simulink subsystem "EMS_sim"  (R2023b)
settings: Solver=VariableStepAuto  StartTime=0.0  StopTime=10.0  RelTol=1e-3
undefined symbols (not defined in the file or in its folder): CH, EMS, Ts
settings Model: Creator=ortolud16324  LastModifiedBy=ortolud16324

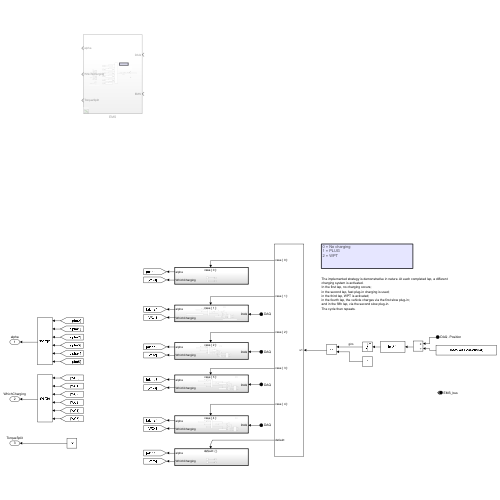
[thumbnail: Simulink's stored preview of the top-level diagram]
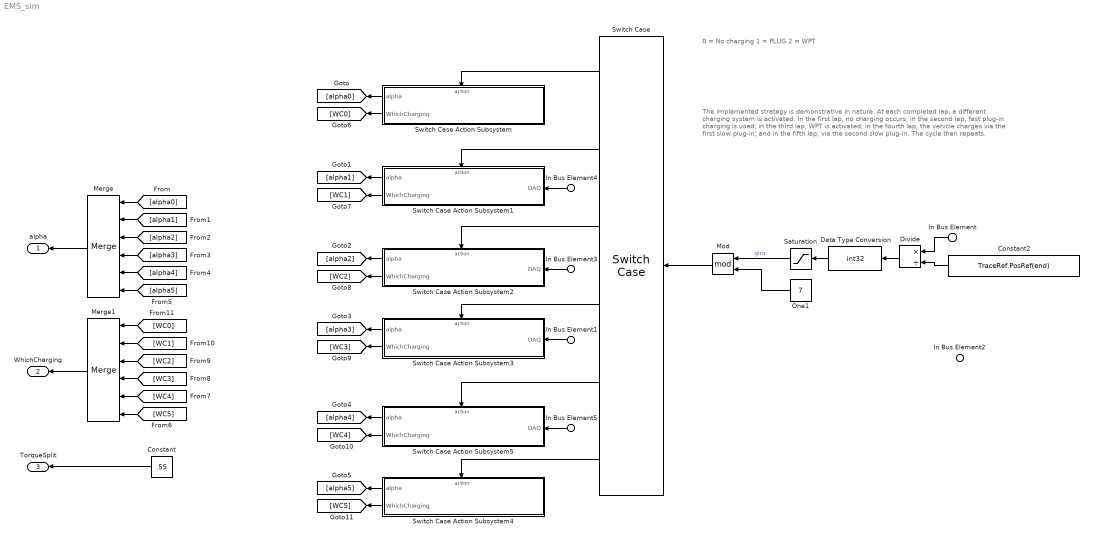
== system EMS_sim ==
  note: 0 = No charging
      | 1 = PLUG
      | 2 = WPT
  note: The implemented strategy is demonstrative in nature. At each completed lap, a different charging system is activated.
      | In the first lap, no charging occurs;
      | in the second lap, fast plug-in charging is used;
      | in the third lap, WPT is activated;
      | in the fourth lap, the vehicle charges via the first slow plug-in;
      | and in the fifth lap, via the second slow plug-in.
      | The cycle then repeats.
  In Bus Element{1,3..5} (4 alike) : Inport  PortName=DAQ
  In Bus Element : Inport  PortName=DAQ  Element=Position
  In Bus Element2 : Inport  Port=2  PortName=EMS_bus
  Constant : Constant  Value=.55  SampleTime=Ts
  Constant2 : Constant  Value=TraceRef.PosRef(end)
  Data Type Conversion : DataTypeConversion  OutDataTypeStr=int32  SaturateOnIntegerOverflow=off  RndMeth=Floor
  Divide : Product  Inputs=*/
  Merge : Merge  Inputs=6
  Merge1 : Merge  Inputs=6
  Mod : Math  Operator=mod
  One1 : Constant  Value=7  OutDataTypeStr=Inherit: Inherit via back propagation
  Saturation : Saturate  UpperLimit=100000  LowerLimit=0
  Switch Case : SwitchCase  CaseConditions={0,1,2,3,4}
  Switch Case Action Subsystem : Subsystem  TreatAsAtomicUnit=on
  Switch Case Action Subsystem1 : Subsystem  TreatAsAtomicUnit=on
  Switch Case Action Subsystem2 : Subsystem  TreatAsAtomicUnit=on
  Switch Case Action Subsystem3 : Subsystem  TreatAsAtomicUnit=on
  Switch Case Action Subsystem4 : Subsystem  TreatAsAtomicUnit=on
  Switch Case Action Subsystem5 : Subsystem  TreatAsAtomicUnit=on
  alpha : Outport
  WhichCharging : Outport  Port=2
  TorqueSplit : Outport  Port=3
  wires:
  Merge1/1 -> WhichCharging/1
  Constant/1 -> TorqueSplit/1
  Merge/1 -> alpha/1
  [alpha2] -> Merge/3
  Switch Case Action Subsystem2/2(WhichCharging) -> [WC2]
  [alpha3] -> Merge/4
  [WC3] -> Merge1/4
  [WC5] -> Merge1/6
  [WC4] -> Merge1/5
  [WC1] -> Merge1/2
  [WC2] -> Merge1/3
  One1/1 -> Mod/2
  In Bus Element5/1 -> Switch Case Action Subsystem5/1(DAQ)
  Switch Case Action Subsystem5/2(WhichCharging) -> [WC4]
  Switch Case/5 -> Switch Case Action Subsystem5/Action
  Switch Case/6 -> Switch Case Action Subsystem4/Action
  [alpha4] -> Merge/5
  Switch Case Action Subsystem2/1(alpha) -> [alpha2]
  Switch Case Action Subsystem3/2(WhichCharging) -> [WC3]
  [alpha0] -> Merge/1
  Switch Case Action Subsystem1/2(WhichCharging) -> [WC1]
  In Bus Element1/1 -> Switch Case Action Subsystem3/1(DAQ)
  Switch Case Action Subsystem5/1(alpha) -> [alpha4]
  Switch Case Action Subsystem3/1(alpha) -> [alpha3]
  Switch Case Action Subsystem/2(WhichCharging) -> [WC0]
  [alpha1] -> Merge/2
  In Bus Element4/1 -> Switch Case Action Subsystem1/1(DAQ)
  Switch Case Action Subsystem/1(alpha) -> [alpha0]
  Switch Case Action Subsystem1/1(alpha) -> [alpha1]
  Switch Case Action Subsystem4/1(alpha) -> [alpha5]
  Data Type Conversion/1 -> Saturation/1
  Mod/1 -> Switch Case/1
  In Bus Element3/1 -> Switch Case Action Subsystem2/1(DAQ)
  Switch Case/4 -> Switch Case Action Subsystem3/Action
  Switch Case/2 -> Switch Case Action Subsystem1/Action
  Switch Case/1 -> Switch Case Action Subsystem/Action
  Divide/1 -> Data Type Conversion/1
  [WC0] -> Merge1/1
  Constant2/1 -> Divide/2
  In Bus Element/1 -> Divide/1
  Saturation/1 -> Mod/1  "giro"
  Switch Case Action Subsystem4/2(WhichCharging) -> [WC5]
  Switch Case/3 -> Switch Case Action Subsystem2/Action
  [alpha5] -> Merge/6

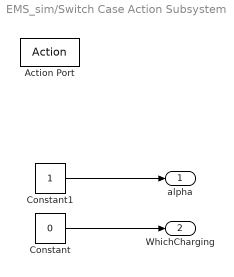
== system EMS_sim/Switch Case Action Subsystem ==
  Action Port : ActionPort
  Constant : Constant  Value=0
  Constant1 : Constant
  alpha : Outport
  WhichCharging : Outport  Port=2
  wires:
  Constant/1 -> WhichCharging/1
  Constant1/1 -> alpha/1

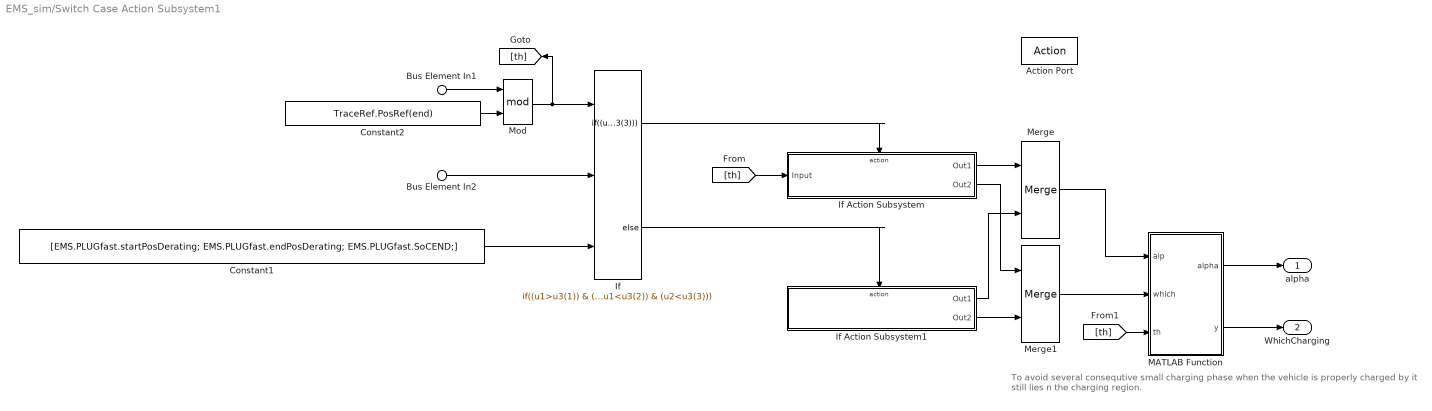
== system EMS_sim/Switch Case Action Subsystem1 ==
  note: To avoid several consequtive small charging phase when the vehicle is properly charged by it still lies n the charging region.
  Bus Element In1 : Inport  PortName=DAQ  Element=Position
  Bus Element In2 : Inport  PortName=DAQ  Element=SoC_BP
  Action Port : ActionPort
  Constant1 : Constant  Value=[EMS.PLUGfast.startPosDerating; EMS.PLUGfast.endPosDerating; EMS.PLUGfast.SoCEND;]
  Constant2 : Constant  Value=TraceRef.PosRef(end)
  If : If  NumInputs=3  IfExpression=(u1>u3(1)) & (u1<u3(2)) & (u2<u3(3))
  If Action Subsystem : Subsystem  TreatAsAtomicUnit=on
  If Action Subsystem1 : Subsystem  TreatAsAtomicUnit=on
  MATLAB Function : MATLAB Function  TreatAsAtomicUnit=on
  Merge : Merge
  Merge1 : Merge
  Mod : Math  Operator=mod
  alpha : Outport
  WhichCharging : Outport  Port=2
  wires:
  Merge/1 -> MATLAB Function/1(alp)
  Merge1/1 -> MATLAB Function/2(which)
  If/1 -> If Action Subsystem/Action
  If/2 -> If Action Subsystem1/Action
  Constant2/1 -> Mod/2
  If Action Subsystem/1(Out1) -> Merge/1
  If Action Subsystem1/1(Out1) -> Merge/2
  Mod/1 -> [th], If/1
  Bus Element In1/1 -> Mod/1
  Bus Element In2/1 -> If/2
  Constant1/1 -> If/3
  If Action Subsystem/2(Out2) -> Merge1/1
  If Action Subsystem1/2(Out2) -> Merge1/2
  [th] -> If Action Subsystem/1(Input)
  MATLAB Function/2(y) -> WhichCharging/1
  [th] -> MATLAB Function/3(th)
  MATLAB Function/1(alpha) -> alpha/1

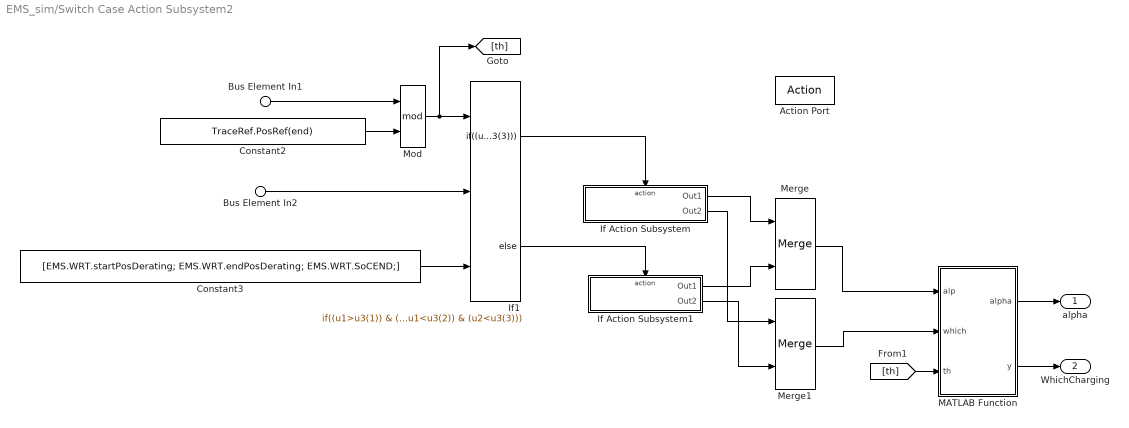
== system EMS_sim/Switch Case Action Subsystem2 ==
  Bus Element In1 : Inport  PortName=DAQ  Element=Position
  Bus Element In2 : Inport  PortName=DAQ  Element=SoC_BP
  Action Port : ActionPort
  Constant2 : Constant  Value=TraceRef.PosRef(end)
  Constant3 : Constant  Value=[EMS.WRT.startPosDerating; EMS.WRT.endPosDerating; EMS.WRT.SoCEND;]
  If Action Subsystem : Subsystem  TreatAsAtomicUnit=on
  If Action Subsystem1 : Subsystem  TreatAsAtomicUnit=on
  If1 : If  NumInputs=3  IfExpression=(u1>u3(1)) & (u1<u3(2)) & (u2<u3(3))
  MATLAB Function : MATLAB Function  TreatAsAtomicUnit=on
  Merge : Merge
  Merge1 : Merge
  Mod : Math  Operator=mod
  alpha : Outport
  WhichCharging : Outport  Port=2
  wires:
  Constant2/1 -> Mod/2
  Mod/1 -> [th], If1/1
  Bus Element In1/1 -> Mod/1
  If1/1 -> If Action Subsystem/Action
  If1/2 -> If Action Subsystem1/Action
  If Action Subsystem/1(Out1) -> Merge/1
  If Action Subsystem1/1(Out1) -> Merge/2
  If Action Subsystem/2(Out2) -> Merge1/1
  If Action Subsystem1/2(Out2) -> Merge1/2
  Bus Element In2/1 -> If1/2
  Constant3/1 -> If1/3
  Merge/1 -> MATLAB Function/1(alp)
  Merge1/1 -> MATLAB Function/2(which)
  [th] -> MATLAB Function/3(th)
  MATLAB Function/1(alpha) -> alpha/1
  MATLAB Function/2(y) -> WhichCharging/1

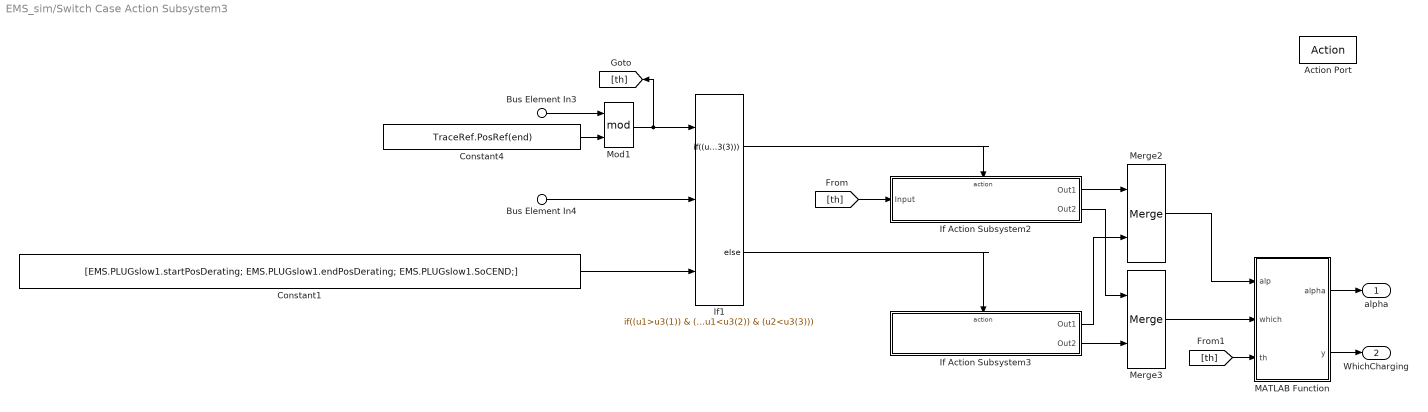
== system EMS_sim/Switch Case Action Subsystem3 ==
  Bus Element In3 : Inport  PortName=DAQ  Element=Position
  Bus Element In4 : Inport  PortName=DAQ  Element=SoC_BP
  Action Port : ActionPort
  Constant1 : Constant  Value=[EMS.PLUGslow1.startPosDerating; EMS.PLUGslow1.endPosDerating; EMS.PLUGslow1.SoCEND;]
  Constant4 : Constant  Value=TraceRef.PosRef(end)
  If Action Subsystem2 : Subsystem  TreatAsAtomicUnit=on
  If Action Subsystem3 : Subsystem  TreatAsAtomicUnit=on
  If1 : If  NumInputs=3  IfExpression=(u1>u3(1)) & (u1<u3(2)) & (u2<u3(3))
  MATLAB Function : MATLAB Function  TreatAsAtomicUnit=on
  Merge2 : Merge
  Merge3 : Merge
  Mod1 : Math  Operator=mod
  alpha : Outport
  WhichCharging : Outport  Port=2
  wires:
  Merge2/1 -> MATLAB Function/1(alp)
  Merge3/1 -> MATLAB Function/2(which)
  If Action Subsystem2/2(Out2) -> Merge3/1
  Constant1/1 -> If1/3
  Bus Element In3/1 -> Mod1/1
  If Action Subsystem2/1(Out1) -> Merge2/1
  Bus Element In4/1 -> If1/2
  Constant4/1 -> Mod1/2
  If Action Subsystem3/1(Out1) -> Merge2/2
  If Action Subsystem3/2(Out2) -> Merge3/2
  [th] -> MATLAB Function/3(th)
  If1/1 -> If Action Subsystem2/Action
  If1/2 -> If Action Subsystem3/Action
  [th] -> If Action Subsystem2/1(Input)
  Mod1/1 -> [th], If1/1
  MATLAB Function/1(alpha) -> alpha/1
  MATLAB Function/2(y) -> WhichCharging/1

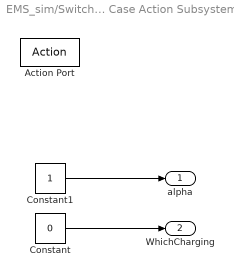
== system EMS_sim/Switch Case Action Subsystem4 ==
  Action Port : ActionPort
  Constant : Constant  Value=0
  Constant1 : Constant
  alpha : Outport
  WhichCharging : Outport  Port=2
  wires:
  Constant/1 -> WhichCharging/1
  Constant1/1 -> alpha/1

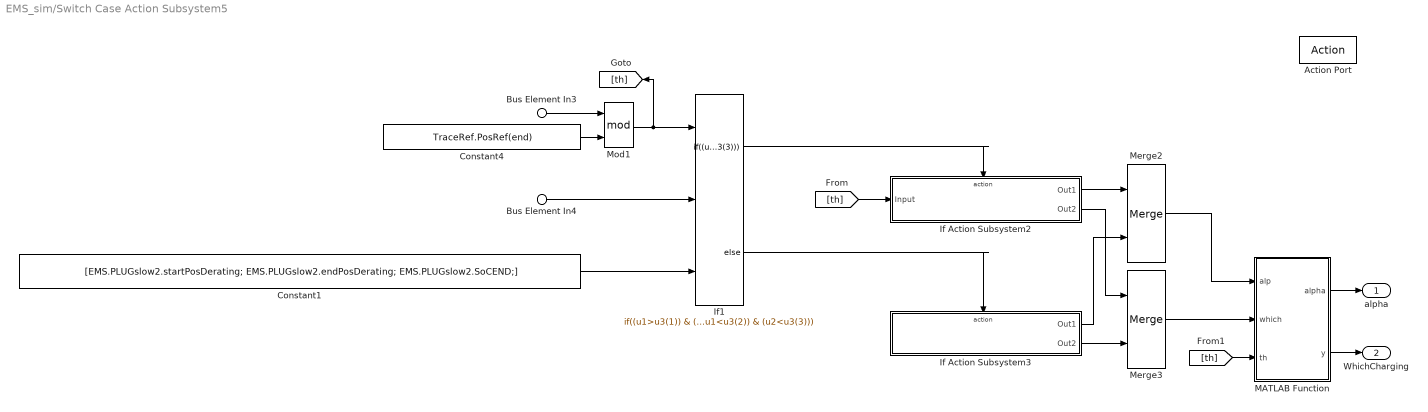
== system EMS_sim/Switch Case Action Subsystem5 ==
  Bus Element In3 : Inport  PortName=DAQ  Element=Position
  Bus Element In4 : Inport  PortName=DAQ  Element=SoC_BP
  Action Port : ActionPort
  Constant1 : Constant  Value=[EMS.PLUGslow2.startPosDerating; EMS.PLUGslow2.endPosDerating; EMS.PLUGslow2.SoCEND;]
  Constant4 : Constant  Value=TraceRef.PosRef(end)
  If Action Subsystem2 : Subsystem  TreatAsAtomicUnit=on
  If Action Subsystem3 : Subsystem  TreatAsAtomicUnit=on
  If1 : If  NumInputs=3  IfExpression=(u1>u3(1)) & (u1<u3(2)) & (u2<u3(3))
  MATLAB Function : MATLAB Function  TreatAsAtomicUnit=on
  Merge2 : Merge
  Merge3 : Merge
  Mod1 : Math  Operator=mod
  alpha : Outport
  WhichCharging : Outport  Port=2
  wires:
  MATLAB Function/2(y) -> WhichCharging/1
  MATLAB Function/1(alpha) -> alpha/1
  Mod1/1 -> If1/1, [th]
  [th] -> If Action Subsystem2/1(Input)
  If1/2 -> If Action Subsystem3/Action
  If1/1 -> If Action Subsystem2/Action
  [th] -> MATLAB Function/3(th)
  If Action Subsystem3/2(Out2) -> Merge3/2
  If Action Subsystem3/1(Out1) -> Merge2/2
  Constant4/1 -> Mod1/2
  Bus Element In4/1 -> If1/2
  If Action Subsystem2/1(Out1) -> Merge2/1
  Bus Element In3/1 -> Mod1/1
  Constant1/1 -> If1/3
  If Action Subsystem2/2(Out2) -> Merge3/1
  Merge3/1 -> MATLAB Function/2(which)
  Merge2/1 -> MATLAB Function/1(alp)

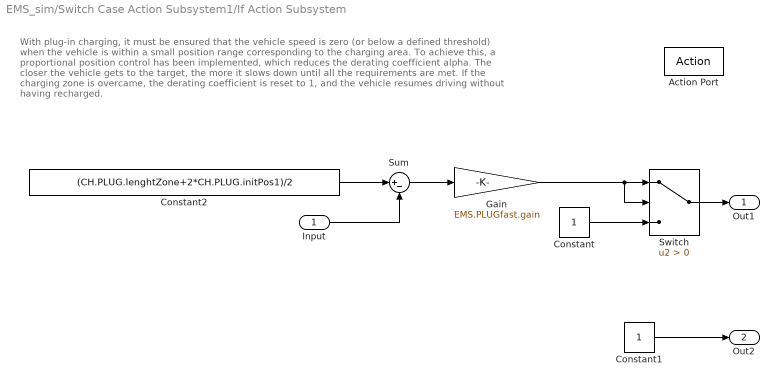
== system EMS_sim/Switch Case Action Subsystem1/If Action Subsystem ==
  note: With plug-in charging, it must be ensured that the vehicle speed is zero (or below a defined
      | threshold) when the vehicle is within a small position range corresponding to the charging
      | area. To achieve this, a proportional position control has been implemented, which reduces
      | the derating coefficient alpha. The closer the vehicle gets to the target, the more it slows
      | down until all the requirements are met.
      | If the charging zone is overcame, the derating coefficient is reset to 1, and the vehicle
      | resumes driving without having recharged.
  Input : Inport
  Action Port : ActionPort
  Constant : Constant
  Constant1 : Constant
  Constant2 : Constant  Value=(CH.PLUG.lenghtZone+2*CH.PLUG.initPos1)/2
  Gain : Gain  Gain=EMS.PLUGfast.gain
  Sum : Sum  Inputs=|+-
  Switch : Switch  Criteria=u2 > Threshold  SaturateOnIntegerOverflow=off  InputSameDT=off
  Out1 : Outport
  Out2 : Outport  Port=2
  wires:
  Constant2/1 -> Sum/1
  Input/1 -> Sum/2
  Switch/1 -> Out1/1
  Constant/1 -> Switch/3
  Sum/1 -> Gain/1
  Gain/1 -> Switch/2, Switch/1
  Constant1/1 -> Out2/1

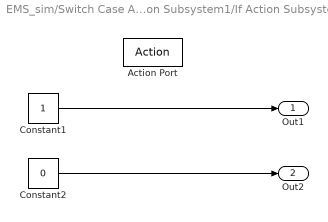
== system EMS_sim/Switch Case Action Subsystem1/If Action Subsystem1 ==
  Action Port : ActionPort
  Constant1 : Constant
  Constant2 : Constant  Value=0
  Out1 : Outport
  Out2 : Outport  Port=2
  wires:
  Constant1/1 -> Out1/1
  Constant2/1 -> Out2/1

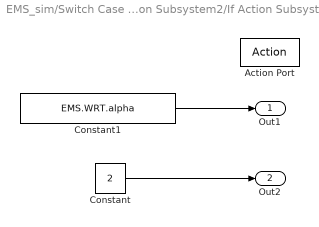
== system EMS_sim/Switch Case Action Subsystem2/If Action Subsystem ==
  Action Port : ActionPort
  Constant : Constant  Value=2
  Constant1 : Constant  Value=EMS.WRT.alpha
  Out1 : Outport
  Out2 : Outport  Port=2
  wires:
  Constant1/1 -> Out1/1
  Constant/1 -> Out2/1

== system EMS_sim/Switch Case Action Subsystem2/If Action Subsystem1 ==
  Action Port : ActionPort
  Constant : Constant  Value=0
  Constant1 : Constant
  Out1 : Outport
  Out2 : Outport  Port=2
  wires:
  Constant1/1 -> Out1/1
  Constant/1 -> Out2/1

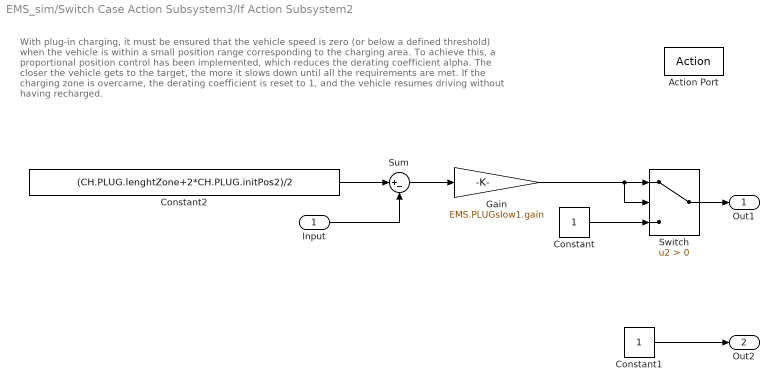
== system EMS_sim/Switch Case Action Subsystem3/If Action Subsystem2 ==
  note: With plug-in charging, it must be ensured that the vehicle speed is zero (or below a defined
      | threshold) when the vehicle is within a small position range corresponding to the charging
      | area. To achieve this, a proportional position control has been implemented, which reduces
      | the derating coefficient alpha. The closer the vehicle gets to the target, the more it slows
      | down until all the requirements are met.
      | If the charging zone is overcame, the derating coefficient is reset to 1, and the vehicle
      | resumes driving without having recharged.
  Input : Inport
  Action Port : ActionPort
  Constant : Constant
  Constant1 : Constant
  Constant2 : Constant  Value=(CH.PLUG.lenghtZone+2*CH.PLUG.initPos2)/2
  Gain : Gain  Gain=EMS.PLUGslow1.gain
  Sum : Sum  Inputs=|+-
  Switch : Switch  Criteria=u2 > Threshold  SaturateOnIntegerOverflow=off  InputSameDT=off
  Out1 : Outport
  Out2 : Outport  Port=2
  wires:
  Constant2/1 -> Sum/1
  Input/1 -> Sum/2
  Switch/1 -> Out1/1
  Constant/1 -> Switch/3
  Sum/1 -> Gain/1
  Gain/1 -> Switch/2, Switch/1
  Constant1/1 -> Out2/1

== system EMS_sim/Switch Case Action Subsystem3/If Action Subsystem3 ==
  Action Port : ActionPort
  Constant1 : Constant
  Constant2 : Constant  Value=0
  Out1 : Outport
  Out2 : Outport  Port=2
  wires:
  Constant1/1 -> Out1/1
  Constant2/1 -> Out2/1

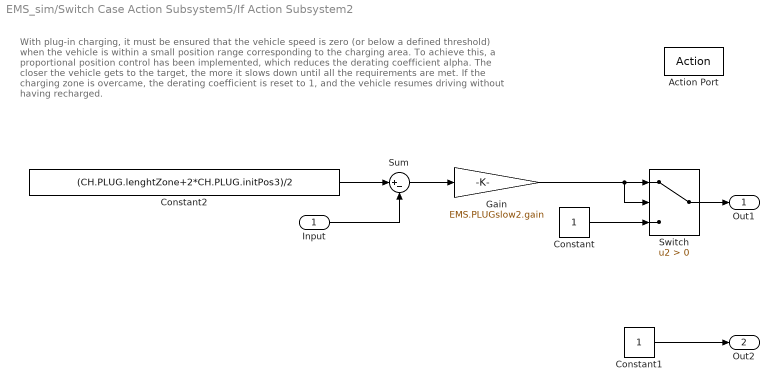
== system EMS_sim/Switch Case Action Subsystem5/If Action Subsystem2 ==
  note: With plug-in charging, it must be ensured that the vehicle speed is zero (or below a defined
      | threshold) when the vehicle is within a small position range corresponding to the charging
      | area. To achieve this, a proportional position control has been implemented, which reduces
      | the derating coefficient alpha. The closer the vehicle gets to the target, the more it slows
      | down until all the requirements are met.
      | If the charging zone is overcame, the derating coefficient is reset to 1, and the vehicle
      | resumes driving without having recharged.
  Input : Inport
  Action Port : ActionPort
  Constant : Constant
  Constant1 : Constant
  Constant2 : Constant  Value=(CH.PLUG.lenghtZone+2*CH.PLUG.initPos3)/2
  Gain : Gain  Gain=EMS.PLUGslow2.gain
  Sum : Sum  Inputs=|+-
  Switch : Switch  Criteria=u2 > Threshold  SaturateOnIntegerOverflow=off  InputSameDT=off
  Out1 : Outport
  Out2 : Outport  Port=2
  wires:
  Constant1/1 -> Out2/1
  Gain/1 -> Switch/1, Switch/2
  Sum/1 -> Gain/1
  Constant/1 -> Switch/3
  Switch/1 -> Out1/1
  Input/1 -> Sum/2
  Constant2/1 -> Sum/1

== system EMS_sim/Switch Case Action Subsystem5/If Action Subsystem3 ==
  Action Port : ActionPort
  Constant1 : Constant
  Constant2 : Constant  Value=0
  Out1 : Outport
  Out2 : Outport  Port=2
  wires:
  Constant2/1 -> Out2/1
  Constant1/1 -> Out1/1

== matlab function EMS_sim/Switch Case Action Subsystem1/MATLAB Function ==
  data: alp input; alpha output; which input; y output; th input; CH parameter
function [alpha,y] = fcn(alp, which, th, CH)

persistent which_km1 dis

if(isempty(which_km1))
    which_km1 = 0;
    dis = 0;
end

y = which;
alpha = alp;

if(((which == 0) && (which_km1 == 1)) || (dis == 1))
    dis = 1;
    y = 0;
    alpha = 1;
end

if (th>(CH.PLUG.initPos1+5))
    dis = 0;
end
    
which_km1 = which;

== matlab function EMS_sim/Switch Case Action Subsystem2/MATLAB Function ==
  data: alp input; alpha output; which input; y output; th input; CH parameter
function [alpha,y] = fcn(alp, which, th, CH)

persistent which_km1 dis

if(isempty(which_km1))
    which_km1 = 0;
    dis = 0;
end

y = which;
alpha = alp;

if(((which == 0) && (which_km1 == 1)) || (dis == 1))
    dis = 1;
    y = 0;
    alpha = 1;
end

if (th>(CH.PLUG.initPos1+5))
    dis = 0;
end
    
which_km1 = which;

== matlab function EMS_sim/Switch Case Action Subsystem3/MATLAB Function ==
  data: alp input; alpha output; which input; y output; th input; CH parameter
function [alpha,y] = fcn(alp, which, th, CH)

persistent which_km1 dis

if(isempty(which_km1))
    which_km1 = 0;
    dis = 0;
end

y = which;
alpha = alp;

if(((which == 0) && (which_km1 == 1)) || (dis == 1))
    dis = 1;
    y = 0;
    alpha = 1;
end

if (th>(CH.PLUG.initPos2+5))
    dis = 0;
end
    
which_km1 = which;

== matlab function EMS_sim/Switch Case Action Subsystem5/MATLAB Function ==
  data: alp input; alpha output; which input; y output; th input; CH parameter
function [alpha,y] = fcn(alp, which, th, CH)

persistent which_km1 dis

if(isempty(which_km1))
    which_km1 = 0;
    dis = 0;
end

y = which;
alpha = alp;

if(((which == 0) && (which_km1 == 1)) || (dis == 1))
    dis = 1;
    y = 0;
    alpha = 1;
end

if (th>(CH.PLUG.initPos3+5))
    dis = 0;
end
    
which_km1 = which;
